simulink subsystem "BatteryHVPackRefSub"  (R2020b)
settings: Solver=VariableStepAuto  StartTime=0.0  StopTime=10.0  RelTol=1e-3
undefined symbols (not defined in the file or in its folder): batteryHV1, batteryHV2
libraries: fl_lib x139, nesl_utility x29, batteryModule_lib x12
(part 2 of 3)

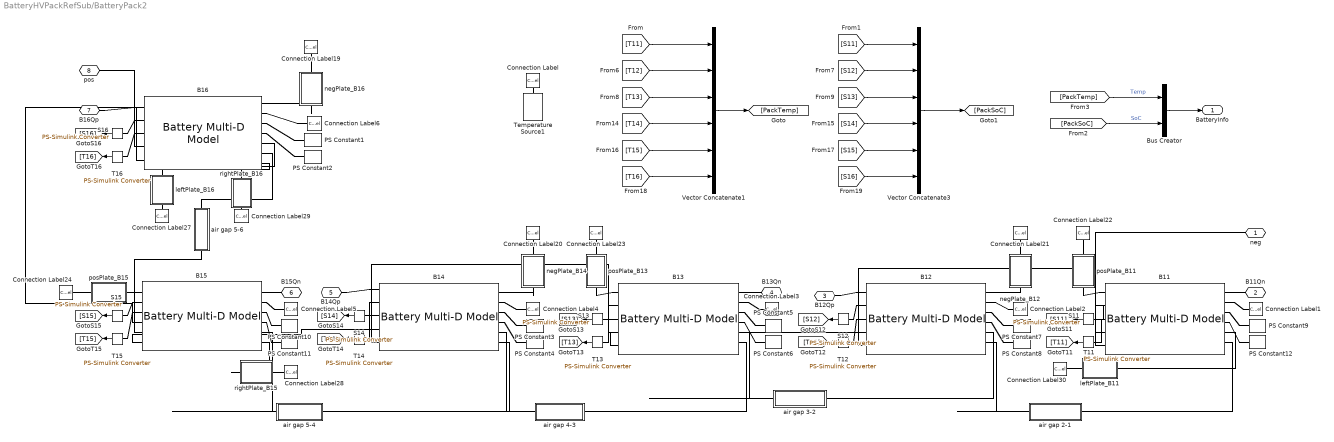
== system BatteryHVPackRefSub/BatteryPack2 ==
  B{11..14} (4 alike) : batteryModule_lib/Battery Multi-D Model  modelComplexity=batteryModule.batteryAbstractionLevel.grouped  thermalManagement=batteryModule.batteryCoolingSystem.thermalPort  thermal_moduleBottom=batteryModule.batteryThermalPortSelection.thermalLUT  thermal_moduleTop=batteryModule.batteryThermalPortSelection.convectionBC  thermal_moduleLeft=batteryModule.batteryThermalPortSelection.thermalPortLumped  thermal_moduleRight=batteryModule.batteryThermalPortSelection.thermalPortLumped  thermal_modulePos=batteryModule.batteryThermalPortSelection.thermalPortLumped  thermal_moduleNeg=batteryModule.batteryThermalPortSelection.thermalPortLumped  Ns=batteryHV2.batteryNs  Np=batteryHV2.batteryNp  cellTypeSelection=batteryModule.batteryTypeSelection.pouch  cellHeight=batteryHV2.batteryCell_H m  cellWidth=batteryHV2.batteryCell_W m  cellThickness=batteryHV2.batteryCell_T m  cellDiameter=0.018 m  cellCylinLine=3  moduleExternalR=batteryHV2.battery_extR Ohm  LUTpointsTemp=batteryHV2.batteryTemp_LUT K  LUTpointsSOC=batteryHV2.batterySOC_LUT  cellAHvector=batteryHV2.batteryCapacity_LUT hr*A  moduleCellAHpercentVar=batteryHV2.batteryModuleCellAhr_ini  cellThermalMass=batteryHV2.batteryCell_mass*batteryHV2.batteryCell_cp J/K  cellThermalCond=batteryHV2.batteryThermal_K1 W/(m*K)  cellThermalCond_inPlane=batteryHV2.batteryThermal_K2 W/(m*K)  cellHeatTrCoeff=1 W/(m^2 * K)  htc_bottom=1 W/(m^2 * K)  htc_top=batteryHV2.batteryModuleTopHTC W/(m^2 * K)  htc_right=1 W/(m^2 * K)  htc_left=1 W/(m^2 * K)  htc_pos=1 W/(m^2 * K)  htc_neg=1 W/(m^2 * K)  cellTemp=batteryHV2.batteryModuleCellT_ini K  cellSOC=batteryHV2.batteryModuleCellSOC_ini  LUTpointsFlowrate_b=batteryHV2.batteryCoolant_flow kg/s  LUTpointsTemp_b=batteryHV2.batteryTemp_LUT K  LUTpointsFlowrate_t=batteryHV2.batteryCoolant_flow kg/s  LUTpointsTemp_t=batteryHV2.batteryTemp_LUT K  LUTpointsFlowrate_r=[.01, .02, .03, .04, .05, .06] kg/s  LUTpointsTemp_r=[273.15, 298.15, 323.15] K  LUTpointsFlowrate_l=[.01, .02, .03, .04, .05, .06] kg/s  LUTpointsTemp_l=[273.15, 298.15, 323.15] K  LUTpointsFlowrate_p=[.01, .02, .03, .04, .05, .06] kg/s  LUTpointsTemp_p=[273.15, 298.15, 323.15] K  LUTpointsFlowrate_n=[.01, .02, .03, .04, .05, .06] kg/s  LUTpointsTemp_n=[273.15, 298.15, 323.15] K  moduleCooling_b=batteryHV2.batteryModuleBottomHTC W/K  moduleCooling_t=batteryHV2.batteryCoolantHTC W/K  moduleCooling_r=zeros(3,6,batteryHV2.batteryNs*batteryHV2.batteryNp) W/K  moduleCooling_l=zeros(3,6,batteryHV2.batteryNs*batteryHV2.batteryNp) W/K  moduleCooling_p=zeros(3,6,batteryHV2.batteryNs*batteryHV2.batteryNp) W/K  moduleCooling_n=zeros(3,6,batteryHV2.batteryNs*batteryHV2.batteryNp) W/K  moduleExtHeat=batteryHV2.batteryModuleExtHeat W  moduleCellBalancing=batteryModule.batteryCellBalancing.none  passiveShuntR=50 Ohm  passiveSWclosedR=0.01 Ohm  passiveSWopenCond=1e-8 1/Ohm  passiveSWthreshold=0.5  prm_dir=ee.enum.battery.prm_dir.noCurrentDirectionality  V0_mat=batteryHV2.batteryEm_LUT V  R0_mat=batteryHV2.batteryR0_LUT Ohm  R0_dis_mat=[.03, .015, .002; .04, .017, .008; .039, .012, .006; .027, .013, .021] Ohm  R0_ch_mat=[.03, .015, .002; .04, .017, .008; .039, .012, .006; .027, .013, .021] Ohm  moduleCellR0PercentVar=batteryHV2.batteryModuleCellR0_ini  prm_leak=ee.enum.battery.prm_leak.disabled  Rleak_vec=[8000, 7000, 6000] Ohm  moduleCellLeakPercentVar=ones(1, 10)  extrapolation_option=ee.enum.extrapolation.nearest  prm_dyn=ee.enum.battery.prm_dyn.rc1  R1_mat=batteryHV2.batteryR1_LUT Ohm  tau1_mat=batteryHV2.batteryTau1_LUT s  R2_mat=[.014, .382, .407; .028, .006, .007; .014, .007, .006; .333, .956, .912] Ohm  tau2_mat=[1, 44, 5644; 11, 24, 506; 2, 14, 330; 3310, 13419, 30216] s  R3_mat=[.014, .382, .407; .028, .006, .007; .014, .007, .006; .333, .956, .912] Ohm  tau3_mat=[1, 44, 5644; 11, 24, 506; 2, 14, 330; 3310, 13419, 30216] s  R4_mat=[.014, .382, .407; .028, .006, .007; .014, .007, .006; .333, .956, .912] Ohm  tau4_mat=[1, 44, 5644; 11, 24, 506; 2, 14, 330; 3310, 13419, 30216] s  R5_mat=[.014, .382, .407; .028, .006, .007; .014, .007, .006; .333, .956, .912] Ohm  tau5_mat=[1, 44, 5644; 11, 24, 506; 2, 14, 330; 3310, 13419, 30216] s  prm_fade=ee.enum.battery.prm_fade.equations  N0=100  dV0=0  dR0=0  dAH=0  dRleak=0  dR1=0  dR2=0  dR3=0  dR4=0  dR5=0  N0vec=[100, 200, 300]  Tfadevec=[298.15, 323.15] K  dV0vec=[0, 0, 0]  dR0vec=[0, 0, 0]  dAHvec=[0, 0, 0]  dRleakvec=[0, 0, 0]  dR1vec=[0, 0, 0]  dR2vec=[0, 0, 0]  dR3vec=[0, 0, 0]  dR4vec=[0, 0, 0]  dR5vec=[0, 0, 0]  dV0mat=[0, 0; 0, 0; 0, 0]  dR0mat=[0, 0; 0, 0; 0, 0]  dAHmat=[0, 0; 0, 0; 0, 0]  dRleakmat=[0, 0; 0, 0; 0, 0]  dR1mat=[0, 0; 0, 0; 0, 0]  dR2mat=[0, 0; 0, 0; 0, 0]  dR3mat=[0, 0; 0, 0; 0, 0]  dR4mat=[0, 0; 0, 0; 0, 0]  dR5mat=[0, 0; 0, 0; 0, 0]
      settings: InternalSimscapePortConfiguration="{\"Bottom\":[{\"id\":\"Ql\",\"label\":\"Ql\",\"type\":\"foundation.thermal.thermal\"},{\"id\":\"Qr\",\"label\":\"Qr\",\"type\":\"foundation.thermal.thermal\"}],\"Left\":[{\"id\":\"Qp\",\"label\":\"Qp\",\"type\":\"foundation.thermal.thermal\"},{\"id\":\"outputCellSOC\",\"label\":\"SOC\",\"type\":\"output\"},{\"id\":\"outputCellTemp\",\"label\":\"Temp\",\"type\":\"output\"}],\"Right\":[{\"id\":\"Qn\",\"label\":\"Qn\",\"type\":\"foundation.thermal.thermal\"},{\"id\":\"H\",\"label\":\"Amb\",\"type\":\"foundation.thermal.thermal\"},{\"id\":\"frac_b\",\"label\":\"FlwR\",\"type\":\"input\"},{\"id\":\"delT_b\",\"label\":\"FlwT\",\"type\":\"input\"}],\"Top\":[{\"id\":\"p\",\"label\":\"pos\",\"type\":\"foundation.electrical.electrical\"},{\"id\":\"n\",\"label\":\"neg\",\"type\":\"foundation.electrical.electrical\"}]}"
  B15 : batteryModule_lib/Battery Multi-D Model  modelComplexity=batteryModule.batteryAbstractionLevel.grouped  thermalManagement=batteryModule.batteryCoolingSystem.thermalPort  thermal_moduleBottom=batteryModule.batteryThermalPortSelection.thermalLUT  thermal_moduleTop=batteryModule.batteryThermalPortSelection.thermalPortLumped  thermal_moduleLeft=batteryModule.batteryThermalPortSelection.thermalPortLumped  thermal_moduleRight=batteryModule.batteryThermalPortSelection.thermalPortLumped  thermal_modulePos=batteryModule.batteryThermalPortSelection.thermalPortLumped  thermal_moduleNeg=batteryModule.batteryThermalPortSelection.thermalPortLumped  Ns=batteryHV2.batteryNs  Np=batteryHV2.batteryNp  cellTypeSelection=batteryModule.batteryTypeSelection.pouch  cellHeight=batteryHV2.batteryCell_H m  cellWidth=batteryHV2.batteryCell_W m  cellThickness=batteryHV2.batteryCell_T m  cellDiameter=0.018 m  cellCylinLine=3  moduleExternalR=batteryHV2.battery_extR Ohm  LUTpointsTemp=batteryHV2.batteryTemp_LUT K  LUTpointsSOC=batteryHV2.batterySOC_LUT  cellAHvector=batteryHV2.batteryCapacity_LUT hr*A  moduleCellAHpercentVar=batteryHV2.batteryModuleCellAhr_ini  cellThermalMass=batteryHV2.batteryCell_mass*batteryHV2.batteryCell_cp J/K  cellThermalCond=batteryHV2.batteryThermal_K1 W/(m*K)  cellThermalCond_inPlane=batteryHV2.batteryThermal_K2 W/(m*K)  cellHeatTrCoeff=1 W/(m^2 * K)  htc_bottom=1 W/(m^2 * K)  htc_top=batteryHV2.batteryModuleTopHTC W/(m^2 * K)  htc_right=1 W/(m^2 * K)  htc_left=1 W/(m^2 * K)  htc_pos=1 W/(m^2 * K)  htc_neg=1 W/(m^2 * K)  cellTemp=batteryHV2.batteryModuleCellT_ini K  cellSOC=batteryHV2.batteryModuleCellSOC_ini  LUTpointsFlowrate_b=batteryHV2.batteryCoolant_flow kg/s  LUTpointsTemp_b=batteryHV2.batteryTemp_LUT K  LUTpointsFlowrate_t=batteryHV2.batteryCoolant_flow kg/s  LUTpointsTemp_t=batteryHV2.batteryTemp_LUT K  LUTpointsFlowrate_r=[.01, .02, .03, .04, .05, .06] kg/s  LUTpointsTemp_r=[273.15, 298.15, 323.15] K  LUTpointsFlowrate_l=[.01, .02, .03, .04, .05, .06] kg/s  LUTpointsTemp_l=[273.15, 298.15, 323.15] K  LUTpointsFlowrate_p=[.01, .02, .03, .04, .05, .06] kg/s  LUTpointsTemp_p=[273.15, 298.15, 323.15] K  LUTpointsFlowrate_n=[.01, .02, .03, .04, .05, .06] kg/s  LUTpointsTemp_n=[273.15, 298.15, 323.15] K  moduleCooling_b=batteryHV2.batteryModuleBottomHTC W/K  moduleCooling_t=batteryHV2.batteryCoolantHTC W/K  moduleCooling_r=zeros(3,6,batteryHV2.batteryNs*batteryHV2.batteryNp) W/K  moduleCooling_l=zeros(3,6,batteryHV2.batteryNs*batteryHV2.batteryNp) W/K  moduleCooling_p=zeros(3,6,batteryHV2.batteryNs*batteryHV2.batteryNp) W/K  moduleCooling_n=zeros(3,6,batteryHV2.batteryNs*batteryHV2.batteryNp) W/K  moduleExtHeat=batteryHV2.batteryModuleExtHeat W  moduleCellBalancing=batteryModule.batteryCellBalancing.none  passiveShuntR=50 Ohm  passiveSWclosedR=0.01 Ohm  passiveSWopenCond=1e-8 1/Ohm  passiveSWthreshold=0.5  prm_dir=ee.enum.battery.prm_dir.noCurrentDirectionality  V0_mat=batteryHV2.batteryEm_LUT V  R0_mat=batteryHV2.batteryR0_LUT Ohm  R0_dis_mat=[.03, .015, .002; .04, .017, .008; .039, .012, .006; .027, .013, .021] Ohm  R0_ch_mat=[.03, .015, .002; .04, .017, .008; .039, .012, .006; .027, .013, .021] Ohm  moduleCellR0PercentVar=batteryHV2.batteryModuleCellR0_ini  prm_leak=ee.enum.battery.prm_leak.disabled  Rleak_vec=[8000, 7000, 6000] Ohm  moduleCellLeakPercentVar=ones(1, 10)  extrapolation_option=ee.enum.extrapolation.nearest  prm_dyn=ee.enum.battery.prm_dyn.rc1  R1_mat=batteryHV2.batteryR1_LUT Ohm  tau1_mat=batteryHV2.batteryTau1_LUT s  R2_mat=[.014, .382, .407; .028, .006, .007; .014, .007, .006; .333, .956, .912] Ohm  tau2_mat=[1, 44, 5644; 11, 24, 506; 2, 14, 330; 3310, 13419, 30216] s  R3_mat=[.014, .382, .407; .028, .006, .007; .014, .007, .006; .333, .956, .912] Ohm  tau3_mat=[1, 44, 5644; 11, 24, 506; 2, 14, 330; 3310, 13419, 30216] s  R4_mat=[.014, .382, .407; .028, .006, .007; .014, .007, .006; .333, .956, .912] Ohm  tau4_mat=[1, 44, 5644; 11, 24, 506; 2, 14, 330; 3310, 13419, 30216] s  R5_mat=[.014, .382, .407; .028, .006, .007; .014, .007, .006; .333, .956, .912] Ohm  tau5_mat=[1, 44, 5644; 11, 24, 506; 2, 14, 330; 3310, 13419, 30216] s  prm_fade=ee.enum.battery.prm_fade.equations  N0=100  dV0=0  dR0=0  dAH=0  dRleak=0  dR1=0  dR2=0  dR3=0  dR4=0  dR5=0  N0vec=[100, 200, 300]  Tfadevec=[298.15, 323.15] K  dV0vec=[0, 0, 0]  dR0vec=[0, 0, 0]  dAHvec=[0, 0, 0]  dRleakvec=[0, 0, 0]  dR1vec=[0, 0, 0]  dR2vec=[0, 0, 0]  dR3vec=[0, 0, 0]  dR4vec=[0, 0, 0]  dR5vec=[0, 0, 0]  dV0mat=[0, 0; 0, 0; 0, 0]  dR0mat=[0, 0; 0, 0; 0, 0]  dAHmat=[0, 0; 0, 0; 0, 0]  dRleakmat=[0, 0; 0, 0; 0, 0]  dR1mat=[0, 0; 0, 0; 0, 0]  dR2mat=[0, 0; 0, 0; 0, 0]  dR3mat=[0, 0; 0, 0; 0, 0]  dR4mat=[0, 0; 0, 0; 0, 0]  dR5mat=[0, 0; 0, 0; 0, 0]
      settings: InternalSimscapePortConfiguration="{\"Bottom\":[{\"id\":\"Ql\",\"label\":\"Ql\",\"type\":\"foundation.thermal.thermal\"},{\"id\":\"Qr\",\"label\":\"Qr\",\"type\":\"foundation.thermal.thermal\"}],\"Left\":[{\"id\":\"Qp\",\"label\":\"Qp\",\"type\":\"foundation.thermal.thermal\"},{\"id\":\"outputCellSOC\",\"label\":\"SOC\",\"type\":\"output\"},{\"id\":\"outputCellTemp\",\"label\":\"Temp\",\"type\":\"output\"}],\"Right\":[{\"id\":\"Qn\",\"label\":\"Qn\",\"type\":\"foundation.thermal.thermal\"},{\"id\":\"H\",\"label\":\"Amb\",\"type\":\"foundation.thermal.thermal\"},{\"id\":\"frac_b\",\"label\":\"FlwR\",\"type\":\"input\"},{\"id\":\"delT_b\",\"label\":\"FlwT\",\"type\":\"input\"}],\"Top\":[{\"id\":\"p\",\"label\":\"pos\",\"type\":\"foundation.electrical.electrical\"},{\"id\":\"Qt\",\"label\":\"Qt\",\"type\":\"foundation.thermal.thermal\"},{\"id\":\"n\",\"label\":\"neg\",\"type\":\"foundation.electrical.electrical\"}]}"
  B16 : batteryModule_lib/Battery Multi-D Model  modelComplexity=batteryModule.batteryAbstractionLevel.grouped  thermalManagement=batteryModule.batteryCoolingSystem.thermalPort  thermal_moduleBottom=batteryModule.batteryThermalPortSelection.thermalPortLumped  thermal_moduleTop=batteryModule.batteryThermalPortSelection.thermalLUT  thermal_moduleLeft=batteryModule.batteryThermalPortSelection.thermalPortLumped  thermal_moduleRight=batteryModule.batteryThermalPortSelection.thermalPortLumped  thermal_modulePos=batteryModule.batteryThermalPortSelection.thermalPortLumped  thermal_moduleNeg=batteryModule.batteryThermalPortSelection.thermalPortLumped  Ns=batteryHV2.batteryNs  Np=batteryHV2.batteryNp  cellTypeSelection=batteryModule.batteryTypeSelection.pouch  cellHeight=batteryHV2.batteryCell_H m  cellWidth=batteryHV2.batteryCell_W m  cellThickness=batteryHV2.batteryCell_T m  cellDiameter=0.018 m  cellCylinLine=3  moduleExternalR=batteryHV2.battery_extR Ohm  LUTpointsTemp=batteryHV2.batteryTemp_LUT K  LUTpointsSOC=batteryHV2.batterySOC_LUT  cellAHvector=batteryHV2.batteryCapacity_LUT hr*A  moduleCellAHpercentVar=batteryHV2.batteryModuleCellAhr_ini  cellThermalMass=batteryHV2.batteryCell_mass*batteryHV2.batteryCell_cp J/K  cellThermalCond=batteryHV2.batteryThermal_K1 W/(m*K)  cellThermalCond_inPlane=batteryHV2.batteryThermal_K2 W/(m*K)  cellHeatTrCoeff=1 W/(m^2 * K)  htc_bottom=1 W/(m^2 * K)  htc_top=batteryHV2.batteryModuleTopHTC W/(m^2 * K)  htc_right=1 W/(m^2 * K)  htc_left=1 W/(m^2 * K)  htc_pos=1 W/(m^2 * K)  htc_neg=1 W/(m^2 * K)  cellTemp=batteryHV2.batteryModuleCellT_ini K  cellSOC=batteryHV2.batteryModuleCellSOC_ini  LUTpointsFlowrate_b=batteryHV2.batteryCoolant_flow kg/s  LUTpointsTemp_b=batteryHV2.batteryTemp_LUT K  LUTpointsFlowrate_t=batteryHV2.batteryCoolant_flow kg/s  LUTpointsTemp_t=batteryHV2.batteryTemp_LUT K  LUTpointsFlowrate_r=[.01, .02, .03, .04, .05, .06] kg/s  LUTpointsTemp_r=[273.15, 298.15, 323.15] K  LUTpointsFlowrate_l=[.01, .02, .03, .04, .05, .06] kg/s  LUTpointsTemp_l=[273.15, 298.15, 323.15] K  LUTpointsFlowrate_p=[.01, .02, .03, .04, .05, .06] kg/s  LUTpointsTemp_p=[273.15, 298.15, 323.15] K  LUTpointsFlowrate_n=[.01, .02, .03, .04, .05, .06] kg/s  LUTpointsTemp_n=[273.15, 298.15, 323.15] K  moduleCooling_b=batteryHV2.batteryModuleBottomHTC W/K  moduleCooling_t=batteryHV2.batteryCoolantHTC W/K  moduleCooling_r=zeros(3,6,batteryHV2.batteryNs*batteryHV2.batteryNp) W/K  moduleCooling_l=zeros(3,6,batteryHV2.batteryNs*batteryHV2.batteryNp) W/K  moduleCooling_p=zeros(3,6,batteryHV2.batteryNs*batteryHV2.batteryNp) W/K  moduleCooling_n=zeros(3,6,batteryHV2.batteryNs*batteryHV2.batteryNp) W/K  moduleExtHeat=batteryHV2.batteryModuleExtHeat W  moduleCellBalancing=batteryModule.batteryCellBalancing.none  passiveShuntR=50 Ohm  passiveSWclosedR=0.01 Ohm  passiveSWopenCond=1e-8 1/Ohm  passiveSWthreshold=0.5  prm_dir=ee.enum.battery.prm_dir.noCurrentDirectionality  V0_mat=batteryHV2.batteryEm_LUT V  R0_mat=batteryHV2.batteryR0_LUT Ohm  R0_dis_mat=[.03, .015, .002; .04, .017, .008; .039, .012, .006; .027, .013, .021] Ohm  R0_ch_mat=[.03, .015, .002; .04, .017, .008; .039, .012, .006; .027, .013, .021] Ohm  moduleCellR0PercentVar=batteryHV2.batteryModuleCellR0_ini  prm_leak=ee.enum.battery.prm_leak.disabled  Rleak_vec=[8000, 7000, 6000] Ohm  moduleCellLeakPercentVar=ones(1, 10)  extrapolation_option=ee.enum.extrapolation.nearest  prm_dyn=ee.enum.battery.prm_dyn.rc1  R1_mat=batteryHV2.batteryR1_LUT Ohm  tau1_mat=batteryHV2.batteryTau1_LUT s  R2_mat=[.014, .382, .407; .028, .006, .007; .014, .007, .006; .333, .956, .912] Ohm  tau2_mat=[1, 44, 5644; 11, 24, 506; 2, 14, 330; 3310, 13419, 30216] s  R3_mat=[.014, .382, .407; .028, .006, .007; .014, .007, .006; .333, .956, .912] Ohm  tau3_mat=[1, 44, 5644; 11, 24, 506; 2, 14, 330; 3310, 13419, 30216] s  R4_mat=[.014, .382, .407; .028, .006, .007; .014, .007, .006; .333, .956, .912] Ohm  tau4_mat=[1, 44, 5644; 11, 24, 506; 2, 14, 330; 3310, 13419, 30216] s  R5_mat=[.014, .382, .407; .028, .006, .007; .014, .007, .006; .333, .956, .912] Ohm  tau5_mat=[1, 44, 5644; 11, 24, 506; 2, 14, 330; 3310, 13419, 30216] s  prm_fade=ee.enum.battery.prm_fade.equations  N0=100  dV0=0  dR0=0  dAH=0  dRleak=0  dR1=0  dR2=0  dR3=0  dR4=0  dR5=0  N0vec=[100, 200, 300]  Tfadevec=[298.15, 323.15] K  dV0vec=[0, 0, 0]  dR0vec=[0, 0, 0]  dAHvec=[0, 0, 0]  dRleakvec=[0, 0, 0]  dR1vec=[0, 0, 0]  dR2vec=[0, 0, 0]  dR3vec=[0, 0, 0]  dR4vec=[0, 0, 0]  dR5vec=[0, 0, 0]  dV0mat=[0, 0; 0, 0; 0, 0]  dR0mat=[0, 0; 0, 0; 0, 0]  dAHmat=[0, 0; 0, 0; 0, 0]  dRleakmat=[0, 0; 0, 0; 0, 0]  dR1mat=[0, 0; 0, 0; 0, 0]  dR2mat=[0, 0; 0, 0; 0, 0]  dR3mat=[0, 0; 0, 0; 0, 0]  dR4mat=[0, 0; 0, 0; 0, 0]  dR5mat=[0, 0; 0, 0; 0, 0]
      settings: InternalSimscapePortConfiguration="{\"Bottom\":[{\"id\":\"Ql\",\"label\":\"Ql\",\"type\":\"foundation.thermal.thermal\"},{\"id\":\"Qb\",\"label\":\"Qb\",\"type\":\"foundation.thermal.thermal\"},{\"id\":\"Qr\",\"label\":\"Qr\",\"type\":\"foundation.thermal.thermal\"}],\"Left\":[{\"id\":\"Qp\",\"label\":\"Qp\",\"type\":\"foundation.thermal.thermal\"},{\"id\":\"outputCellSOC\",\"label\":\"SOC\",\"type\":\"output\"},{\"id\":\"outputCellTemp\",\"label\":\"Temp\",\"type\":\"output\"}],\"Right\":[{\"id\":\"Qn\",\"label\":\"Qn\",\"type\":\"foundation.thermal.thermal\"},{\"id\":\"H\",\"label\":\"Amb\",\"type\":\"foundation.thermal.thermal\"},{\"id\":\"frac_t\",\"label\":\"FlwR\",\"type\":\"input\"},{\"id\":\"delT_t\",\"label\":\"FlwT\",\"type\":\"input\"}],\"Top\":[{\"id\":\"p\",\"label\":\"pos\",\"type\":\"foundation.electrical.electrical\"},{\"id\":\"n\",\"label\":\"neg\",\"type\":\"foundation.electrical.electrical\"}]}"
  Bus Creator : BusCreator  Inputs=2
  Connection Label{,1..6,19..24,27..30} (17 alike) : ConnectionLabel  Label=Amb
  PS Constant{1,3,5,7,9..10} (6 alike) : fl_lib/Physical Signals/Sources/PS Constant  constant=batteryHV.batteryCoolantFlwR
  PS Constant{2,4,6,8,11..12} (6 alike) : fl_lib/Physical Signals/Sources/PS Constant  constant=batteryHV.batteryCoolantFlwT K
  S{11..16} (6 alike) : nesl_utility/PS-Simulink Converter  PhysicalDomain=network_engine_domain  SubClassName=ps_output  LeftPortType=input  RightPortType=output  PseudoPeriodic=off  Frequencies=[]  Unit=1  AffineConversion=off
      settings: SourceProductBaseCode=PW,SS
  T{11..16} (6 alike) : nesl_utility/PS-Simulink Converter  PhysicalDomain=network_engine_domain  SubClassName=ps_output  LeftPortType=input  RightPortType=output  PseudoPeriodic=off  Frequencies=[]  Unit=K  AffineConversion=off
      settings: SourceProductBaseCode=PW,SS
  Temperature Source1 : fl_lib/Thermal/Thermal Sources/Temperature Source  temperature=batteryHV.AmbTemp K
  Vector Concatenate1 : Concatenate  NumInputs=6
  Vector Concatenate3 : Concatenate  NumInputs=6
  air gap 2-1 : Subsystem
  air gap 3-2 : Subsystem
  air gap 4-3 : Subsystem
  air gap 5-4 : Subsystem
  air gap 5-6 : Subsystem
  leftPlate_B11 : Subsystem
  leftPlate_B16 : Subsystem
  negPlate_B12 : Subsystem
  negPlate_B14 : Subsystem
  negPlate_B16 : Subsystem
  posPlate_B11 : Subsystem
  posPlate_B13 : Subsystem
  posPlate_B15 : Subsystem
  rightPlate_B15 : Subsystem
  rightPlate_B16 : Subsystem
  neg : PMIOPort  Side=Left
  B11Qn : PMIOPort  Port=2  Side=Left
  B12Qp : PMIOPort  Port=3  Side=Left
  B13Qn : PMIOPort  Port=4  Side=Left
  B14Qp : PMIOPort  Port=5  Side=Left
  B15Qn : PMIOPort  Port=6  Side=Left
  B16Qp : PMIOPort  Port=7  Side=Left
  pos : PMIOPort  Port=8  Side=Right
  BatteryInfo : Outport
  wires:
  [PackTemp] -> Bus Creator/1  "Temp"
  [PackSoC] -> Bus Creator/2  "SoC"
  Bus Creator/1 -> BatteryInfo/1
  S16/1 -> [S16]
  [S12] -> Vector Concatenate3/2
  [T16] -> Vector Concatenate1/6
  [S13] -> Vector Concatenate3/3
  [T12] -> Vector Concatenate1/2
  [T13] -> Vector Concatenate1/3
  [T15] -> Vector Concatenate1/5
  [T11] -> Vector Concatenate1/1
  [T14] -> Vector Concatenate1/4
  [S14] -> Vector Concatenate3/4
  Vector Concatenate3/1 -> [PackSoC]
  Vector Concatenate1/1 -> [PackTemp]
  [S11] -> Vector Concatenate3/1
  [S15] -> Vector Concatenate3/5
  [S16] -> Vector Concatenate3/6
  T15/1 -> [T15]
  S15/1 -> [S15]
  S14/1 -> [S14]
  T13/1 -> [T13]
  T14/1 -> [T14]
  T11/1 -> [T11]
  T12/1 -> [T12]
  S12/1 -> [S12]
  S13/1 -> [S13]
  S11/1 -> [S11]
  T16/1 -> [T16]
  connections:
  air gap 2-1/RConn1 -- B11/RConn6
  air gap 3-2/RConn1 -- B12/RConn5
  air gap 4-3/RConn1 -- B13/RConn6
  air gap 5-4/RConn1 -- B14/RConn5
  PS Constant12/RConn1 -- B11/RConn4
  PS Constant9/RConn1 -- B11/RConn3
  PS Constant8/RConn1 -- B12/RConn4
  PS Constant7/RConn1 -- B12/RConn3
  PS Constant5/RConn1 -- B13/RConn3
  PS Constant6/RConn1 -- B13/RConn4
  PS Constant4/RConn1 -- B14/RConn4
  PS Constant3/RConn1 -- B14/RConn3
  PS Constant11/RConn1 -- B15/RConn4
  PS Constant10/RConn1 -- B15/RConn3
  PS Constant2/RConn1 -- B16/RConn4
  PS Constant1/RConn1 -- B16/RConn3
  Connection Label/LConn1 -- Temperature Source1/LConn1
  B12/LConn1 -- B12Qp/RConn1
  B16/LConn4 -- pos/RConn1
  B14/LConn1 -- B14Qp/RConn1
  B13/RConn1 -- B13Qn/RConn1
  B11/RConn1 -- B11Qn/RConn1
  B16/LConn2 -- S16/LConn1
  B11/LConn5 -- neg/RConn1
  B16/LConn1 -- B16Qp/RConn1
  posPlate_B11/LConn1 -- Connection Label22/LConn1
  air gap 3-2/LConn1 -- B13/RConn5
  B12/LConn4 -- B13/LConn5
  B14/LConn3 -- T14/LConn1
  B13/LConn2 -- S13/LConn1
  B12/LConn2 -- S12/LConn1
  air gap 4-3/LConn1 -- B14/RConn6
  B12/RConn2 -- Connection Label2/LConn1
  B11/LConn3 -- T11/LConn1
  B11/LConn4 -- B12/LConn5
  B12/LConn3 -- T12/LConn1
  Connection Label6/LConn1 -- B16/RConn2
  posPlate_B13/RConn1 -- B13/LConn1
  rightPlate_B16/RConn1 -- B16/RConn7
  B15/RConn1 -- B15Qn/RConn1
  B11/LConn2 -- S11/LConn1
  Connection Label29/LConn1 -- rightPlate_B16/LConn1
  rightPlate_B15/RConn1 -- B15/RConn6
  B15/LConn4 -- B16/LConn5
  air gap 2-1/LConn1 -- B12/RConn6
  rightPlate_B15/LConn1 -- Connection Label28/LConn1
  B13/RConn2 -- Connection Label3/LConn1
  posPlate_B13/LConn1 -- Connection Label23/LConn1
  B13/LConn3 -- T13/LConn1
  B11/RConn2 -- Connection Label1/LConn1
  air gap 5-6/RConn1 -- B16/RConn6
  posPlate_B11/RConn1 -- B11/LConn1
  Connection Label24/LConn1 -- posPlate_B15/LConn1
  B15/LConn6 -- B14/LConn4
  B15/LConn3 -- T15/LConn1
  posPlate_B15/RConn1 -- B15/LConn1
  B15/LConn2 -- S15/LConn1
  Connection Label4/LConn1 -- B14/RConn2
  air gap 5-6/LConn1 -- B15/LConn5
  B13/LConn4 -- B14/LConn5
  air gap 5-4/LConn1 -- B15/RConn5
  Connection Label5/LConn1 -- B15/RConn2
  B14/LConn2 -- S14/LConn1
  B16/LConn3 -- T16/LConn1
  negPlate_B16/RConn1 -- B16/RConn1
  negPlate_B16/LConn1 -- Connection Label19/LConn1
  Connection Label27/LConn1 -- leftPlate_B16/LConn1
  leftPlate_B16/RConn1 -- B16/RConn5
  negPlate_B14/RConn1 -- B14/RConn1
  negPlate_B14/LConn1 -- Connection Label20/LConn1
  B12/RConn1 -- negPlate_B12/RConn1
  negPlate_B12/LConn1 -- Connection Label21/LConn1
  Connection Label30/LConn1 -- leftPlate_B11/LConn1
  leftPlate_B11/RConn1 -- B11/RConn5

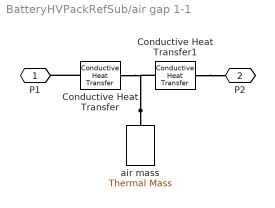
== system BatteryHVPackRefSub/air gap 1-1 ==
  Conductive Heat Transfer : fl_lib/Thermal/Thermal Elements/Conductive Heat Transfer  area=batteryHV1.batteryCell_H*batteryHV1.batteryCell_W m^2  thickness=0.002 m  th_cond=0.024 W/(m*K)  T_specify=off  T_priority=None  T=0 K  T_nominal_specify=off  T_nominal_unit=K  T_nominal_value=1  Q_specify=off  Q_priority=None  Q=0 W  Q_nominal_specify=off  Q_nominal_unit=W  Q_nominal_value=1
  Conductive Heat Transfer1 : fl_lib/Thermal/Thermal Elements/Conductive Heat Transfer  area=batteryHV2.batteryCell_H*batteryHV2.batteryCell_W m^2  thickness=0.002 m  th_cond=0.024 W/(m*K)  T_specify=off  T_priority=None  T=0 K  T_nominal_specify=off  T_nominal_unit=K  T_nominal_value=1  Q_specify=off  Q_priority=None  Q=0 W  Q_nominal_specify=off  Q_nominal_unit=W  Q_nominal_value=1
  air mass : fl_lib/Thermal/Thermal Elements/Thermal Mass  mass=batteryHV1.batteryCell_H*batteryHV1.batteryCell_W*0.002*1.28 kg  sp_heat=1000 J/kg/K  T_specify=off  T_priority=High  T=300 K  T_nominal_specify=off  T_nominal_unit=K  T_nominal_value=1  Q_specify=off  Q_priority=None  Q=0 W  Q_nominal_specify=off  Q_nominal_unit=W  Q_nominal_value=1
  P1 : PMIOPort  Side=Left
  P2 : PMIOPort  Port=2  Side=Right
  connections:
  Conductive Heat Transfer/LConn1 -- P1/RConn1
  Conductive Heat Transfer1/RConn1 -- P2/RConn1
  air mass/LConn1 -- Conductive Heat Transfer/RConn1 -- Conductive Heat Transfer1/LConn1

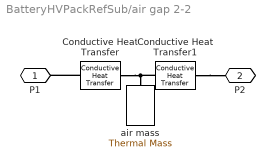
== system BatteryHVPackRefSub/air gap 2-2 ==
  Conductive Heat Transfer : fl_lib/Thermal/Thermal Elements/Conductive Heat Transfer  area=batteryHV1.batteryCell_H*batteryHV1.batteryCell_W m^2  thickness=0.002 m  th_cond=0.024 W/(m*K)  T_specify=off  T_priority=None  T=0 K  T_nominal_specify=off  T_nominal_unit=K  T_nominal_value=1  Q_specify=off  Q_priority=None  Q=0 W  Q_nominal_specify=off  Q_nominal_unit=W  Q_nominal_value=1
  Conductive Heat Transfer1 : fl_lib/Thermal/Thermal Elements/Conductive Heat Transfer  area=batteryHV2.batteryCell_H*batteryHV2.batteryCell_W m^2  thickness=0.002 m  th_cond=0.024 W/(m*K)  T_specify=off  T_priority=None  T=0 K  T_nominal_specify=off  T_nominal_unit=K  T_nominal_value=1  Q_specify=off  Q_priority=None  Q=0 W  Q_nominal_specify=off  Q_nominal_unit=W  Q_nominal_value=1
  air mass : fl_lib/Thermal/Thermal Elements/Thermal Mass  mass=batteryHV1.batteryCell_H*batteryHV1.batteryCell_W*0.002*1.28 kg  sp_heat=1000 J/kg/K  T_specify=off  T_priority=High  T=300 K  T_nominal_specify=off  T_nominal_unit=K  T_nominal_value=1  Q_specify=off  Q_priority=None  Q=0 W  Q_nominal_specify=off  Q_nominal_unit=W  Q_nominal_value=1
  P1 : PMIOPort  Side=Left
  P2 : PMIOPort  Port=2  Side=Right
  connections:
  Conductive Heat Transfer1/LConn1 -- Conductive Heat Transfer/RConn1 -- air mass/LConn1
  Conductive Heat Transfer1/RConn1 -- P2/RConn1
  Conductive Heat Transfer/LConn1 -- P1/RConn1

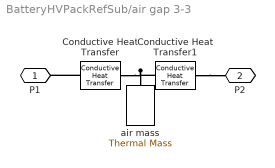
== system BatteryHVPackRefSub/air gap 3-3 ==
  Conductive Heat Transfer : fl_lib/Thermal/Thermal Elements/Conductive Heat Transfer  area=batteryHV1.batteryCell_H*batteryHV1.batteryCell_W m^2  thickness=0.002 m  th_cond=0.024 W/(m*K)  T_specify=off  T_priority=None  T=0 K  T_nominal_specify=off  T_nominal_unit=K  T_nominal_value=1  Q_specify=off  Q_priority=None  Q=0 W  Q_nominal_specify=off  Q_nominal_unit=W  Q_nominal_value=1
  Conductive Heat Transfer1 : fl_lib/Thermal/Thermal Elements/Conductive Heat Transfer  area=batteryHV2.batteryCell_H*batteryHV2.batteryCell_W m^2  thickness=0.002 m  th_cond=0.024 W/(m*K)  T_specify=off  T_priority=None  T=0 K  T_nominal_specify=off  T_nominal_unit=K  T_nominal_value=1  Q_specify=off  Q_priority=None  Q=0 W  Q_nominal_specify=off  Q_nominal_unit=W  Q_nominal_value=1
  air mass : fl_lib/Thermal/Thermal Elements/Thermal Mass  mass=batteryHV1.batteryCell_H*batteryHV1.batteryCell_W*0.002*1.28 kg  sp_heat=1000 J/kg/K  T_specify=off  T_priority=High  T=300 K  T_nominal_specify=off  T_nominal_unit=K  T_nominal_value=1  Q_specify=off  Q_priority=None  Q=0 W  Q_nominal_specify=off  Q_nominal_unit=W  Q_nominal_value=1
  P1 : PMIOPort  Side=Left
  P2 : PMIOPort  Port=2  Side=Right
  connections:
  Conductive Heat Transfer/LConn1 -- P1/RConn1
  Conductive Heat Transfer1/RConn1 -- P2/RConn1
  air mass/LConn1 -- Conductive Heat Transfer/RConn1 -- Conductive Heat Transfer1/LConn1

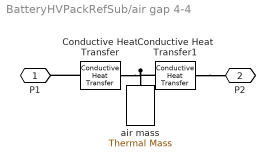
== system BatteryHVPackRefSub/air gap 4-4 ==
  Conductive Heat Transfer : fl_lib/Thermal/Thermal Elements/Conductive Heat Transfer  area=batteryHV1.batteryCell_H*batteryHV1.batteryCell_W m^2  thickness=0.002 m  th_cond=0.024 W/(m*K)  T_specify=off  T_priority=None  T=0 K  T_nominal_specify=off  T_nominal_unit=K  T_nominal_value=1  Q_specify=off  Q_priority=None  Q=0 W  Q_nominal_specify=off  Q_nominal_unit=W  Q_nominal_value=1
  Conductive Heat Transfer1 : fl_lib/Thermal/Thermal Elements/Conductive Heat Transfer  area=batteryHV2.batteryCell_H*batteryHV2.batteryCell_W m^2  thickness=0.002 m  th_cond=0.024 W/(m*K)  T_specify=off  T_priority=None  T=0 K  T_nominal_specify=off  T_nominal_unit=K  T_nominal_value=1  Q_specify=off  Q_priority=None  Q=0 W  Q_nominal_specify=off  Q_nominal_unit=W  Q_nominal_value=1
  air mass : fl_lib/Thermal/Thermal Elements/Thermal Mass  mass=batteryHV1.batteryCell_H*batteryHV1.batteryCell_W*0.002*1.28 kg  sp_heat=1000 J/kg/K  T_specify=off  T_priority=High  T=300 K  T_nominal_specify=off  T_nominal_unit=K  T_nominal_value=1  Q_specify=off  Q_priority=None  Q=0 W  Q_nominal_specify=off  Q_nominal_unit=W  Q_nominal_value=1
  P1 : PMIOPort  Side=Left
  P2 : PMIOPort  Port=2  Side=Right
  connections:
  Conductive Heat Transfer/LConn1 -- P1/RConn1
  Conductive Heat Transfer1/RConn1 -- P2/RConn1
  air mass/LConn1 -- Conductive Heat Transfer/RConn1 -- Conductive Heat Transfer1/LConn1

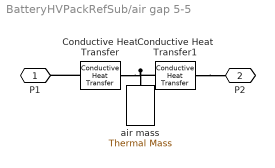
== system BatteryHVPackRefSub/air gap 5-5 ==
  Conductive Heat Transfer : fl_lib/Thermal/Thermal Elements/Conductive Heat Transfer  area=batteryHV1.batteryCell_H*batteryHV1.batteryCell_W m^2  thickness=0.002 m  th_cond=0.024 W/(m*K)  T_specify=off  T_priority=None  T=0 K  T_nominal_specify=off  T_nominal_unit=K  T_nominal_value=1  Q_specify=off  Q_priority=None  Q=0 W  Q_nominal_specify=off  Q_nominal_unit=W  Q_nominal_value=1
  Conductive Heat Transfer1 : fl_lib/Thermal/Thermal Elements/Conductive Heat Transfer  area=batteryHV2.batteryCell_H*batteryHV2.batteryCell_W m^2  thickness=0.002 m  th_cond=0.024 W/(m*K)  T_specify=off  T_priority=None  T=0 K  T_nominal_specify=off  T_nominal_unit=K  T_nominal_value=1  Q_specify=off  Q_priority=None  Q=0 W  Q_nominal_specify=off  Q_nominal_unit=W  Q_nominal_value=1
  air mass : fl_lib/Thermal/Thermal Elements/Thermal Mass  mass=batteryHV1.batteryCell_H*batteryHV1.batteryCell_W*0.002*1.28 kg  sp_heat=1000 J/kg/K  T_specify=off  T_priority=High  T=300 K  T_nominal_specify=off  T_nominal_unit=K  T_nominal_value=1  Q_specify=off  Q_priority=None  Q=0 W  Q_nominal_specify=off  Q_nominal_unit=W  Q_nominal_value=1
  P1 : PMIOPort  Side=Left
  P2 : PMIOPort  Port=2  Side=Right
  connections:
  Conductive Heat Transfer/LConn1 -- P1/RConn1
  Conductive Heat Transfer1/RConn1 -- P2/RConn1
  air mass/LConn1 -- Conductive Heat Transfer/RConn1 -- Conductive Heat Transfer1/LConn1

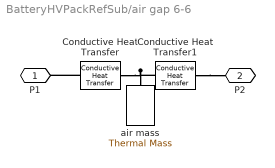
== system BatteryHVPackRefSub/air gap 6-6 ==
  Conductive Heat Transfer : fl_lib/Thermal/Thermal Elements/Conductive Heat Transfer  area=batteryHV1.batteryCell_H*batteryHV1.batteryCell_W m^2  thickness=0.002 m  th_cond=0.024 W/(m*K)  T_specify=off  T_priority=None  T=0 K  T_nominal_specify=off  T_nominal_unit=K  T_nominal_value=1  Q_specify=off  Q_priority=None  Q=0 W  Q_nominal_specify=off  Q_nominal_unit=W  Q_nominal_value=1
  Conductive Heat Transfer1 : fl_lib/Thermal/Thermal Elements/Conductive Heat Transfer  area=batteryHV2.batteryCell_H*batteryHV2.batteryCell_W m^2  thickness=0.002 m  th_cond=0.024 W/(m*K)  T_specify=off  T_priority=None  T=0 K  T_nominal_specify=off  T_nominal_unit=K  T_nominal_value=1  Q_specify=off  Q_priority=None  Q=0 W  Q_nominal_specify=off  Q_nominal_unit=W  Q_nominal_value=1
  air mass : fl_lib/Thermal/Thermal Elements/Thermal Mass  mass=batteryHV1.batteryCell_H*batteryHV1.batteryCell_W*0.002*1.28 kg  sp_heat=1000 J/kg/K  T_specify=off  T_priority=High  T=300 K  T_nominal_specify=off  T_nominal_unit=K  T_nominal_value=1  Q_specify=off  Q_priority=None  Q=0 W  Q_nominal_specify=off  Q_nominal_unit=W  Q_nominal_value=1
  P1 : PMIOPort  Side=Left
  P2 : PMIOPort  Port=2  Side=Right
  connections:
  Conductive Heat Transfer/LConn1 -- P1/RConn1
  Conductive Heat Transfer1/RConn1 -- P2/RConn1
  air mass/LConn1 -- Conductive Heat Transfer/RConn1 -- Conductive Heat Transfer1/LConn1

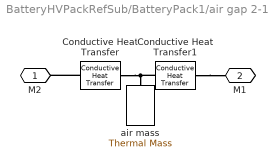
== system BatteryHVPackRefSub/BatteryPack1/air gap 2-1 ==
  Conductive Heat Transfer : fl_lib/Thermal/Thermal Elements/Conductive Heat Transfer  area=batteryHV1.batteryCell_T*batteryHV1.battery_N_cells*batteryHV1.batteryCell_H m^2  thickness=0.002 m  th_cond=0.024 W/(m*K)  T_specify=off  T_priority=None  T=0 K  T_nominal_specify=off  T_nominal_unit=K  T_nominal_value=1  Q_specify=off  Q_priority=None  Q=0 W  Q_nominal_specify=off  Q_nominal_unit=W  Q_nominal_value=1
  Conductive Heat Transfer1 : fl_lib/Thermal/Thermal Elements/Conductive Heat Transfer  area=batteryHV1.batteryCell_H*batteryHV1.batteryCell_H m^2  thickness=0.002 m  th_cond=0.024 W/(m*K)  T_specify=off  T_priority=None  T=0 K  T_nominal_specify=off  T_nominal_unit=K  T_nominal_value=1  Q_specify=off  Q_priority=None  Q=0 W  Q_nominal_specify=off  Q_nominal_unit=W  Q_nominal_value=1
  air mass : fl_lib/Thermal/Thermal Elements/Thermal Mass  mass=batteryHV1.batteryCell_H*batteryHV1.batteryCell_T*batteryHV1.battery_N_cells*0.002*1.28 kg  sp_heat=1000 J/kg/K  T_specify=off  T_priority=High  T=300 K  T_nominal_specify=off  T_nominal_unit=K  T_nominal_value=1  Q_specify=off  Q_priority=None  Q=0 W  Q_nominal_specify=off  Q_nominal_unit=W  Q_nominal_value=1
  M2 : PMIOPort  Side=Left
  M1 : PMIOPort  Port=2  Side=Right
  connections:
  Conductive Heat Transfer1/LConn1 -- Conductive Heat Transfer/RConn1 -- air mass/LConn1
  Conductive Heat Transfer1/RConn1 -- M1/RConn1
  Conductive Heat Transfer/LConn1 -- M2/RConn1

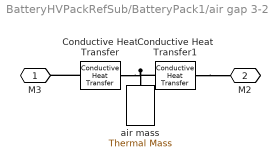
== system BatteryHVPackRefSub/BatteryPack1/air gap 3-2 ==
  Conductive Heat Transfer : fl_lib/Thermal/Thermal Elements/Conductive Heat Transfer  area=batteryHV1.batteryCell_T*batteryHV1.battery_N_cells*batteryHV1.batteryCell_H m^2  thickness=0.002 m  th_cond=0.024 W/(m*K)  T_specify=off  T_priority=None  T=0 K  T_nominal_specify=off  T_nominal_unit=K  T_nominal_value=1  Q_specify=off  Q_priority=None  Q=0 W  Q_nominal_specify=off  Q_nominal_unit=W  Q_nominal_value=1
  Conductive Heat Transfer1 : fl_lib/Thermal/Thermal Elements/Conductive Heat Transfer  area=batteryHV1.batteryCell_H*batteryHV1.batteryCell_H m^2  thickness=0.002 m  th_cond=0.024 W/(m*K)  T_specify=off  T_priority=None  T=0 K  T_nominal_specify=off  T_nominal_unit=K  T_nominal_value=1  Q_specify=off  Q_priority=None  Q=0 W  Q_nominal_specify=off  Q_nominal_unit=W  Q_nominal_value=1
  air mass : fl_lib/Thermal/Thermal Elements/Thermal Mass  mass=batteryHV1.batteryCell_H*batteryHV1.batteryCell_T*batteryHV1.battery_N_cells*0.002*1.28 kg  sp_heat=1000 J/kg/K  T_specify=off  T_priority=High  T=300 K  T_nominal_specify=off  T_nominal_unit=K  T_nominal_value=1  Q_specify=off  Q_priority=None  Q=0 W  Q_nominal_specify=off  Q_nominal_unit=W  Q_nominal_value=1
  M3 : PMIOPort  Side=Left
  M2 : PMIOPort  Port=2  Side=Right
  connections:
  Conductive Heat Transfer/LConn1 -- M3/RConn1
  Conductive Heat Transfer1/RConn1 -- M2/RConn1
  air mass/LConn1 -- Conductive Heat Transfer/RConn1 -- Conductive Heat Transfer1/LConn1

== system BatteryHVPackRefSub/BatteryPack1/air gap 4-3 ==
  Conductive Heat Transfer : fl_lib/Thermal/Thermal Elements/Conductive Heat Transfer  area=batteryHV1.batteryCell_T*batteryHV1.battery_N_cells*batteryHV1.batteryCell_H m^2  thickness=0.002 m  th_cond=0.024 W/(m*K)  T_specify=off  T_priority=None  T=0 K  T_nominal_specify=off  T_nominal_unit=K  T_nominal_value=1  Q_specify=off  Q_priority=None  Q=0 W  Q_nominal_specify=off  Q_nominal_unit=W  Q_nominal_value=1
  Conductive Heat Transfer1 : fl_lib/Thermal/Thermal Elements/Conductive Heat Transfer  area=batteryHV1.batteryCell_H*batteryHV1.batteryCell_H m^2  thickness=0.002 m  th_cond=0.024 W/(m*K)  T_specify=off  T_priority=None  T=0 K  T_nominal_specify=off  T_nominal_unit=K  T_nominal_value=1  Q_specify=off  Q_priority=None  Q=0 W  Q_nominal_specify=off  Q_nominal_unit=W  Q_nominal_value=1
  air mass : fl_lib/Thermal/Thermal Elements/Thermal Mass  mass=batteryHV1.batteryCell_H*batteryHV1.batteryCell_T*batteryHV1.battery_N_cells*0.002*1.28 kg  sp_heat=1000 J/kg/K  T_specify=off  T_priority=High  T=300 K  T_nominal_specify=off  T_nominal_unit=K  T_nominal_value=1  Q_specify=off  Q_priority=None  Q=0 W  Q_nominal_specify=off  Q_nominal_unit=W  Q_nominal_value=1
  M4 : PMIOPort  Side=Left
  M3 : PMIOPort  Port=2  Side=Right
  connections:
  Conductive Heat Transfer1/LConn1 -- Conductive Heat Transfer/RConn1 -- air mass/LConn1
  Conductive Heat Transfer1/RConn1 -- M3/RConn1
  Conductive Heat Transfer/LConn1 -- M4/RConn1

== system BatteryHVPackRefSub/BatteryPack1/air gap 5-4 ==
  Conductive Heat Transfer : fl_lib/Thermal/Thermal Elements/Conductive Heat Transfer  area=batteryHV1.batteryCell_T*batteryHV1.battery_N_cells*batteryHV1.batteryCell_H m^2  thickness=0.002 m  th_cond=0.024 W/(m*K)  T_specify=off  T_priority=None  T=0 K  T_nominal_specify=off  T_nominal_unit=K  T_nominal_value=1  Q_specify=off  Q_priority=None  Q=0 W  Q_nominal_specify=off  Q_nominal_unit=W  Q_nominal_value=1
  Conductive Heat Transfer1 : fl_lib/Thermal/Thermal Elements/Conductive Heat Transfer  area=batteryHV1.batteryCell_H*batteryHV1.batteryCell_H m^2  thickness=0.002 m  th_cond=0.024 W/(m*K)  T_specify=off  T_priority=None  T=0 K  T_nominal_specify=off  T_nominal_unit=K  T_nominal_value=1  Q_specify=off  Q_priority=None  Q=0 W  Q_nominal_specify=off  Q_nominal_unit=W  Q_nominal_value=1
  air mass : fl_lib/Thermal/Thermal Elements/Thermal Mass  mass=batteryHV1.batteryCell_H*batteryHV1.batteryCell_T*batteryHV1.battery_N_cells*0.002*1.28 kg  sp_heat=1000 J/kg/K  T_specify=off  T_priority=High  T=300 K  T_nominal_specify=off  T_nominal_unit=K  T_nominal_value=1  Q_specify=off  Q_priority=None  Q=0 W  Q_nominal_specify=off  Q_nominal_unit=W  Q_nominal_value=1
  M5 : PMIOPort  Side=Left
  M4 : PMIOPort  Port=2  Side=Right
  connections:
  Conductive Heat Transfer/LConn1 -- M5/RConn1
  Conductive Heat Transfer1/RConn1 -- M4/RConn1
  air mass/LConn1 -- Conductive Heat Transfer/RConn1 -- Conductive Heat Transfer1/LConn1

== system BatteryHVPackRefSub/BatteryPack1/air gap 5-6 ==
  Conductive Heat Transfer : fl_lib/Thermal/Thermal Elements/Conductive Heat Transfer  area=batteryHV1.batteryCell_T*batteryHV1.battery_N_cells*batteryHV1.batteryCell_W m^2  thickness=0.002 m  th_cond=0.024 W/(m*K)  T_specify=off  T_priority=None  T=0 K  T_nominal_specify=off  T_nominal_unit=K  T_nominal_value=1  Q_specify=off  Q_priority=None  Q=0 W  Q_nominal_specify=off  Q_nominal_unit=W  Q_nominal_value=1
  Conductive Heat Transfer1 : fl_lib/Thermal/Thermal Elements/Conductive Heat Transfer  area=batteryHV1.batteryCell_H*batteryHV1.batteryCell_W m^2  thickness=0.002 m  th_cond=0.024 W/(m*K)  T_specify=off  T_priority=None  T=0 K  T_nominal_specify=off  T_nominal_unit=K  T_nominal_value=1  Q_specify=off  Q_priority=None  Q=0 W  Q_nominal_specify=off  Q_nominal_unit=W  Q_nominal_value=1
  air mass : fl_lib/Thermal/Thermal Elements/Thermal Mass  mass=batteryHV1.batteryCell_W*batteryHV1.batteryCell_T*batteryHV1.battery_N_cells*0.002*1.28 kg  sp_heat=1000 J/kg/K  T_specify=off  T_priority=High  T=300 K  T_nominal_specify=off  T_nominal_unit=K  T_nominal_value=1  Q_specify=off  Q_priority=None  Q=0 W  Q_nominal_specify=off  Q_nominal_unit=W  Q_nominal_value=1
  M5 : PMIOPort  Side=Left
  M6 : PMIOPort  Port=2  Side=Right
  connections:
  Conductive Heat Transfer1/LConn1 -- Conductive Heat Transfer/RConn1 -- air mass/LConn1
  Conductive Heat Transfer1/RConn1 -- M6/RConn1
  Conductive Heat Transfer/LConn1 -- M5/RConn1

== system BatteryHVPackRefSub/BatteryPack1/leftPlate_B11 ==
  Conductive Heat Transfer : fl_lib/Thermal/Thermal Elements/Conductive Heat Transfer  area=batteryHV1.batteryCell_H*batteryHV1.batteryCell_T*batteryHV1.battery_N_cells m^2  thickness=0.002 m  th_cond=0.024 W/(m*K)  T_specify=off  T_priority=None  T=0 K  T_nominal_specify=off  T_nominal_unit=K  T_nominal_value=1  Q_specify=off  Q_priority=None  Q=0 W  Q_nominal_specify=off  Q_nominal_unit=W  Q_nominal_value=1
  Conductive Heat Transfer1 : fl_lib/Thermal/Thermal Elements/Conductive Heat Transfer  area=batteryHV1.batteryCell_H*batteryHV1.batteryCell_T*batteryHV1.battery_N_cells m^2  thickness=0.002 m  th_cond=0.024 W/(m*K)  T_specify=off  T_priority=None  T=0 K  T_nominal_specify=off  T_nominal_unit=K  T_nominal_value=1  Q_specify=off  Q_priority=None  Q=0 W  Q_nominal_specify=off  Q_nominal_unit=W  Q_nominal_value=1
  plasticPlate : fl_lib/Thermal/Thermal Elements/Thermal Mass  mass=batteryHV1.batteryCell_H*batteryHV1.batteryCell_T*batteryHV1.battery_N_cells*0.002*44 kg  sp_heat=400 J/kg/K  T_specify=off  T_priority=High  T=300 K  T_nominal_specify=off  T_nominal_unit=K  T_nominal_value=1  Q_specify=off  Q_priority=None  Q=0 W  Q_nominal_specify=off  Q_nominal_unit=W  Q_nominal_value=1
  amb : PMIOPort  Side=Left
  M : PMIOPort  Port=2  Side=Right
  connections:
  Conductive Heat Transfer1/RConn1 -- amb/RConn1
  Conductive Heat Transfer/LConn1 -- M/RConn1
  plasticPlate/LConn1 -- Conductive Heat Transfer/RConn1 -- Conductive Heat Transfer1/LConn1

== system BatteryHVPackRefSub/BatteryPack1/leftPlate_B16 ==
  Conductive Heat Transfer : fl_lib/Thermal/Thermal Elements/Conductive Heat Transfer  area=batteryHV1.batteryCell_H*batteryHV1.batteryCell_T*batteryHV1.battery_N_cells m^2  thickness=0.002 m  th_cond=0.024 W/(m*K)  T_specify=off  T_priority=None  T=0 K  T_nominal_specify=off  T_nominal_unit=K  T_nominal_value=1  Q_specify=off  Q_priority=None  Q=0 W  Q_nominal_specify=off  Q_nominal_unit=W  Q_nominal_value=1
  Conductive Heat Transfer1 : fl_lib/Thermal/Thermal Elements/Conductive Heat Transfer  area=batteryHV1.batteryCell_H*batteryHV1.batteryCell_T*batteryHV1.battery_N_cells m^2  thickness=0.002 m  th_cond=0.024 W/(m*K)  T_specify=off  T_priority=None  T=0 K  T_nominal_specify=off  T_nominal_unit=K  T_nominal_value=1  Q_specify=off  Q_priority=None  Q=0 W  Q_nominal_specify=off  Q_nominal_unit=W  Q_nominal_value=1
  plasticPlate : fl_lib/Thermal/Thermal Elements/Thermal Mass  mass=batteryHV1.batteryCell_H*batteryHV1.batteryCell_T*batteryHV1.battery_N_cells*0.002*44 kg  sp_heat=400 J/kg/K  T_specify=off  T_priority=High  T=300 K  T_nominal_specify=off  T_nominal_unit=K  T_nominal_value=1  Q_specify=off  Q_priority=None  Q=0 W  Q_nominal_specify=off  Q_nominal_unit=W  Q_nominal_value=1
  amb : PMIOPort  Side=Left
  M : PMIOPort  Port=2  Side=Right
  connections:
  Conductive Heat Transfer1/RConn1 -- amb/RConn1
  Conductive Heat Transfer/LConn1 -- M/RConn1
  plasticPlate/LConn1 -- Conductive Heat Transfer/RConn1 -- Conductive Heat Transfer1/LConn1

== system BatteryHVPackRefSub/BatteryPack1/negPlate_B12 ==
  Conductive Heat Transfer : fl_lib/Thermal/Thermal Elements/Conductive Heat Transfer  area=batteryHV1.batteryCell_H*batteryHV1.batteryCell_W m^2  thickness=0.002 m  th_cond=0.024 W/(m*K)  T_specify=off  T_priority=None  T=0 K  T_nominal_specify=off  T_nominal_unit=K  T_nominal_value=1  Q_specify=off  Q_priority=None  Q=0 W  Q_nominal_specify=off  Q_nominal_unit=W  Q_nominal_value=1
  Conductive Heat Transfer1 : fl_lib/Thermal/Thermal Elements/Conductive Heat Transfer  area=batteryHV1.batteryCell_H*batteryHV1.batteryCell_W m^2  thickness=0.002 m  th_cond=0.024 W/(m*K)  T_specify=off  T_priority=None  T=0 K  T_nominal_specify=off  T_nominal_unit=K  T_nominal_value=1  Q_specify=off  Q_priority=None  Q=0 W  Q_nominal_specify=off  Q_nominal_unit=W  Q_nominal_value=1
  plasticPlate : fl_lib/Thermal/Thermal Elements/Thermal Mass  mass=batteryHV1.batteryCell_H*batteryHV1.batteryCell_T*batteryHV1.battery_N_cells*0.002*44 kg  sp_heat=400 J/kg/K  T_specify=off  T_priority=High  T=300 K  T_nominal_specify=off  T_nominal_unit=K  T_nominal_value=1  Q_specify=off  Q_priority=None  Q=0 W  Q_nominal_specify=off  Q_nominal_unit=W  Q_nominal_value=1
  amb : PMIOPort  Side=Left
  M : PMIOPort  Port=2  Side=Right
  connections:
  Conductive Heat Transfer1/LConn1 -- Conductive Heat Transfer/RConn1 -- plasticPlate/LConn1
  Conductive Heat Transfer/LConn1 -- M/RConn1
  Conductive Heat Transfer1/RConn1 -- amb/RConn1

== system BatteryHVPackRefSub/BatteryPack1/negPlate_B14 ==
  Conductive Heat Transfer : fl_lib/Thermal/Thermal Elements/Conductive Heat Transfer  area=batteryHV1.batteryCell_H*batteryHV1.batteryCell_W m^2  thickness=0.002 m  th_cond=0.024 W/(m*K)  T_specify=off  T_priority=None  T=0 K  T_nominal_specify=off  T_nominal_unit=K  T_nominal_value=1  Q_specify=off  Q_priority=None  Q=0 W  Q_nominal_specify=off  Q_nominal_unit=W  Q_nominal_value=1
  Conductive Heat Transfer1 : fl_lib/Thermal/Thermal Elements/Conductive Heat Transfer  area=batteryHV1.batteryCell_H*batteryHV1.batteryCell_W m^2  thickness=0.002 m  th_cond=0.024 W/(m*K)  T_specify=off  T_priority=None  T=0 K  T_nominal_specify=off  T_nominal_unit=K  T_nominal_value=1  Q_specify=off  Q_priority=None  Q=0 W  Q_nominal_specify=off  Q_nominal_unit=W  Q_nominal_value=1
  plasticPlate : fl_lib/Thermal/Thermal Elements/Thermal Mass  mass=batteryHV1.batteryCell_H*batteryHV1.batteryCell_T*batteryHV1.battery_N_cells*0.002*44 kg  sp_heat=400 J/kg/K  T_specify=off  T_priority=High  T=300 K  T_nominal_specify=off  T_nominal_unit=K  T_nominal_value=1  Q_specify=off  Q_priority=None  Q=0 W  Q_nominal_specify=off  Q_nominal_unit=W  Q_nominal_value=1
  amb : PMIOPort  Side=Left
  M : PMIOPort  Port=2  Side=Right
  connections:
  Conductive Heat Transfer1/LConn1 -- Conductive Heat Transfer/RConn1 -- plasticPlate/LConn1
  Conductive Heat Transfer/LConn1 -- M/RConn1
  Conductive Heat Transfer1/RConn1 -- amb/RConn1

== system BatteryHVPackRefSub/BatteryPack1/negPlate_B16 ==
  Conductive Heat Transfer : fl_lib/Thermal/Thermal Elements/Conductive Heat Transfer  area=batteryHV1.batteryCell_H*batteryHV1.batteryCell_W m^2  thickness=0.002 m  th_cond=0.024 W/(m*K)  T_specify=off  T_priority=None  T=0 K  T_nominal_specify=off  T_nominal_unit=K  T_nominal_value=1  Q_specify=off  Q_priority=None  Q=0 W  Q_nominal_specify=off  Q_nominal_unit=W  Q_nominal_value=1
  Conductive Heat Transfer1 : fl_lib/Thermal/Thermal Elements/Conductive Heat Transfer  area=batteryHV1.batteryCell_H*batteryHV1.batteryCell_W m^2  thickness=0.002 m  th_cond=0.024 W/(m*K)  T_specify=off  T_priority=None  T=0 K  T_nominal_specify=off  T_nominal_unit=K  T_nominal_value=1  Q_specify=off  Q_priority=None  Q=0 W  Q_nominal_specify=off  Q_nominal_unit=W  Q_nominal_value=1
  plasticPlate : fl_lib/Thermal/Thermal Elements/Thermal Mass  mass=batteryHV1.batteryCell_H*batteryHV1.batteryCell_T*batteryHV1.battery_N_cells*0.002*44 kg  sp_heat=400 J/kg/K  T_specify=off  T_priority=High  T=300 K  T_nominal_specify=off  T_nominal_unit=K  T_nominal_value=1  Q_specify=off  Q_priority=None  Q=0 W  Q_nominal_specify=off  Q_nominal_unit=W  Q_nominal_value=1
  amb : PMIOPort  Side=Left
  M : PMIOPort  Port=2  Side=Right
  connections:
  Conductive Heat Transfer1/RConn1 -- amb/RConn1
  Conductive Heat Transfer/LConn1 -- M/RConn1
  plasticPlate/LConn1 -- Conductive Heat Transfer/RConn1 -- Conductive Heat Transfer1/LConn1

== system BatteryHVPackRefSub/BatteryPack1/posPlate_B11 ==
  Conductive Heat Transfer : fl_lib/Thermal/Thermal Elements/Conductive Heat Transfer  area=batteryHV1.batteryCell_H*batteryHV1.batteryCell_W m^2  thickness=0.002 m  th_cond=0.024 W/(m*K)  T_specify=off  T_priority=None  T=0 K  T_nominal_specify=off  T_nominal_unit=K  T_nominal_value=1  Q_specify=off  Q_priority=None  Q=0 W  Q_nominal_specify=off  Q_nominal_unit=W  Q_nominal_value=1
  Conductive Heat Transfer1 : fl_lib/Thermal/Thermal Elements/Conductive Heat Transfer  area=batteryHV1.batteryCell_H*batteryHV1.batteryCell_W m^2  thickness=0.002 m  th_cond=0.024 W/(m*K)  T_specify=off  T_priority=None  T=0 K  T_nominal_specify=off  T_nominal_unit=K  T_nominal_value=1  Q_specify=off  Q_priority=None  Q=0 W  Q_nominal_specify=off  Q_nominal_unit=W  Q_nominal_value=1
  plasticPlate : fl_lib/Thermal/Thermal Elements/Thermal Mass  mass=batteryHV1.batteryCell_H*batteryHV1.batteryCell_T*batteryHV1.battery_N_cells*0.002*44 kg  sp_heat=400 J/kg/K  T_specify=off  T_priority=High  T=300 K  T_nominal_specify=off  T_nominal_unit=K  T_nominal_value=1  Q_specify=off  Q_priority=None  Q=0 W  Q_nominal_specify=off  Q_nominal_unit=W  Q_nominal_value=1
  amb : PMIOPort  Side=Left
  M : PMIOPort  Port=2  Side=Right
  connections:
  Conductive Heat Transfer1/RConn1 -- amb/RConn1
  Conductive Heat Transfer/LConn1 -- M/RConn1
  plasticPlate/LConn1 -- Conductive Heat Transfer/RConn1 -- Conductive Heat Transfer1/LConn1

== system BatteryHVPackRefSub/BatteryPack1/posPlate_B13 ==
  Conductive Heat Transfer : fl_lib/Thermal/Thermal Elements/Conductive Heat Transfer  area=batteryHV1.batteryCell_H*batteryHV1.batteryCell_W m^2  thickness=0.002 m  th_cond=0.024 W/(m*K)  T_specify=off  T_priority=None  T=0 K  T_nominal_specify=off  T_nominal_unit=K  T_nominal_value=1  Q_specify=off  Q_priority=None  Q=0 W  Q_nominal_specify=off  Q_nominal_unit=W  Q_nominal_value=1
  Conductive Heat Transfer1 : fl_lib/Thermal/Thermal Elements/Conductive Heat Transfer  area=batteryHV1.batteryCell_H*batteryHV1.batteryCell_W m^2  thickness=0.002 m  th_cond=0.024 W/(m*K)  T_specify=off  T_priority=None  T=0 K  T_nominal_specify=off  T_nominal_unit=K  T_nominal_value=1  Q_specify=off  Q_priority=None  Q=0 W  Q_nominal_specify=off  Q_nominal_unit=W  Q_nominal_value=1
  plasticPlate : fl_lib/Thermal/Thermal Elements/Thermal Mass  mass=batteryHV1.batteryCell_H*batteryHV1.batteryCell_T*batteryHV1.battery_N_cells*0.002*44 kg  sp_heat=400 J/kg/K  T_specify=off  T_priority=High  T=300 K  T_nominal_specify=off  T_nominal_unit=K  T_nominal_value=1  Q_specify=off  Q_priority=None  Q=0 W  Q_nominal_specify=off  Q_nominal_unit=W  Q_nominal_value=1
  amb : PMIOPort  Side=Left
  M : PMIOPort  Port=2  Side=Right
  connections:
  Conductive Heat Transfer1/RConn1 -- amb/RConn1
  Conductive Heat Transfer/LConn1 -- M/RConn1
  plasticPlate/LConn1 -- Conductive Heat Transfer/RConn1 -- Conductive Heat Transfer1/LConn1
